simulink model "dtmp_analysis"  (R2025b)
settings: Solver=ode23tb  StartTime=0.0  StopTime=simlength  FixedStep=tc  MaxStep=tc  RelTol=1e-3
values from neighbouring files (symbols this model uses):
  dT_base = 0.4e-3    (= 0.0004)    [init_dtmp_analysis.m]
  N = 40    [init_dtmp_analysis.m]
  tau_dt = Rdt*Cdt    (= 2.706e-06)    [init_dtmp_analysis.m]
  tau_mp = Rmp*Cmp    (= 8.91e-07)    [init_dtmp_analysis.m]
  tc = 1e-7    (= 1e-07)    [init_dtg.m]    (also in init_dtmp_analysis.m)
  Ton_base = 0.333e-6    (= 3.33e-07)    [init_dtmp_analysis.m]
  vin_cmd = 12    [init_dtg.m]    (also in init_dtmp_analysis.m = 15)
libraries: deadtime_with_minimum_pulse_generator x5
settings Model: SimulationMode=accelerator  Creator=dbagn  LastModifiedBy=ltnbda
settings DataIOCC: SaveOutput=off  SignalLogging=off  DSMLogging=off  SaveTime=off  ReturnWorkspaceOutputs=off

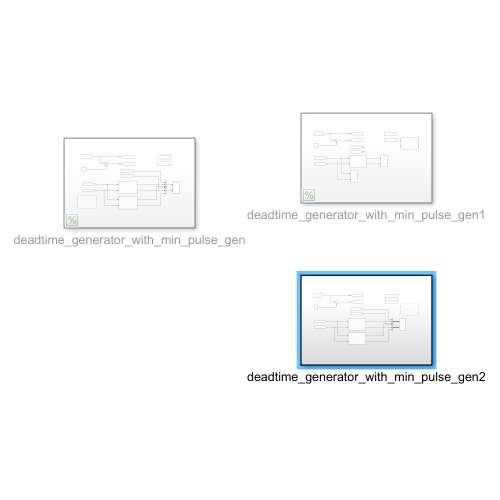
[thumbnail: Simulink's stored preview of the top-level diagram]
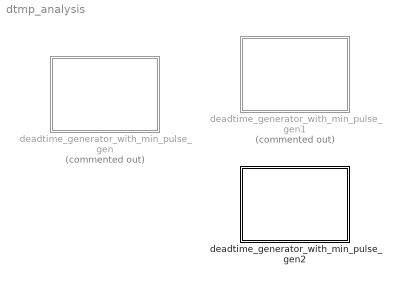
== system dtmp_analysis ==
  deadtime_generator_with_min_pulse_gen : Subsystem  Commented=on
  deadtime_generator_with_min_pulse_gen1 : Subsystem  Commented=on
  deadtime_generator_with_min_pulse_gen2 : Subsystem

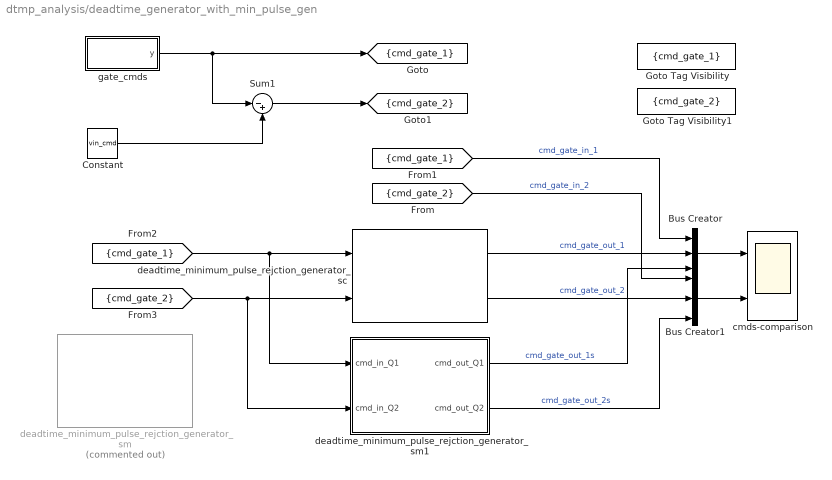
== system dtmp_analysis/deadtime_generator_with_min_pulse_gen ==
  Bus Creator : BusCreator  Inputs=3
  Bus Creator1 : BusCreator  Inputs=3
  Constant : Constant  Value=vin_cmd
  Goto Tag Visibility : GotoTagVisibility  GotoTag=cmd_gate_1
  Goto Tag Visibility1 : GotoTagVisibility  GotoTag=cmd_gate_2
  Sum1 : Sum  Inputs=|-+
  cmds-comparison : Scope  NumInputPorts=2
      settings: SampleTime=tc  ActiveDisplayYMinimum=-1.8749999999999996  ActiveDisplayYMaximum=16.875
  deadtime_minimum_pulse_rejction_generator_sc : deadtime_with_minimum_pulse_generator/deadtime_minimum_pulse_rejction_generator_sc  Vpos_rail_dtg=15  Vneg_rail_dtg=0  Cdt=Cdt  Rdt=Rdt  Cmp=Cmp  Rmp=Rmp
  deadtime_minimum_pulse_rejction_generator_sm : deadtime_with_minimum_pulse_generator/deadtime_minimum_pulse_rejction_generator_sm  Commented=on  Vpos_rail_dtg=12  deadtime=2e-6  minimum_pulse=2e-6
  deadtime_minimum_pulse_rejction_generator_sm1 : Subsystem  mask{Vpos_rail_dtg=15, deadtime=tau_dt, minimum_pulse=tau_mp, tc_m=tc}
      mask prompts: Vpos_rail_dtg "Positive Voltage Rail Supply"; deadtime "DeadTime [s]"; minimum_pulse "Minimum Pulse [s]"; tc_m "tc [s]"
  gate_cmds : Subsystem
  tag scope: cmd_gate_1=scoped, cmd_gate_2=scoped
  wires:
  gate_cmds/1(y) -> [cmd_gate_1], Sum1/1
  [cmd_gate_2] -> Bus Creator1/1  "cmd_gate_in_2"
  [cmd_gate_1] -> Bus Creator/1  "cmd_gate_in_1"
  deadtime_minimum_pulse_rejction_generator_sc/2 -> Bus Creator1/2  "cmd_gate_out_2"
  deadtime_minimum_pulse_rejction_generator_sc/1 -> Bus Creator/2  "cmd_gate_out_1"
  Constant/1 -> Sum1/2
  Sum1/1 -> [cmd_gate_2]
  Bus Creator/1 -> cmds-comparison/1
  Bus Creator1/1 -> cmds-comparison/2
  [cmd_gate_1] -> deadtime_minimum_pulse_rejction_generator_sm1/1(cmd_in_Q1), deadtime_minimum_pulse_rejction_generator_sc/1
  [cmd_gate_2] -> deadtime_minimum_pulse_rejction_generator_sm1/2(cmd_in_Q2), deadtime_minimum_pulse_rejction_generator_sc/2
  deadtime_minimum_pulse_rejction_generator_sm1/1(cmd_out_Q1) -> Bus Creator/3  "cmd_gate_out_1s"
  deadtime_minimum_pulse_rejction_generator_sm1/2(cmd_out_Q2) -> Bus Creator1/3  "cmd_gate_out_2s"

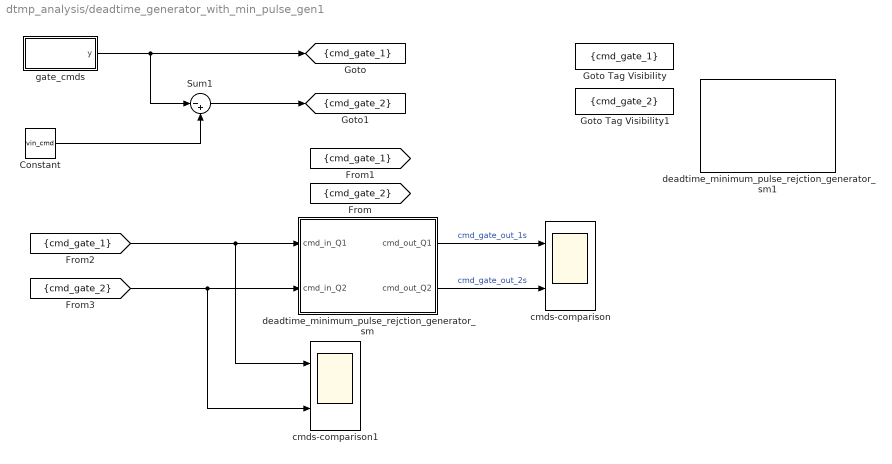
== system dtmp_analysis/deadtime_generator_with_min_pulse_gen1 ==
  Constant : Constant  Value=vin_cmd
  Goto Tag Visibility : GotoTagVisibility  GotoTag=cmd_gate_1
  Goto Tag Visibility1 : GotoTagVisibility  GotoTag=cmd_gate_2
  Sum1 : Sum  Inputs=|-+
  cmds-comparison : Scope  NumInputPorts=2
      settings: SampleTime=tc  ActiveDisplayYMinimum=-1.8749999999999996  ActiveDisplayYMaximum=16.875
  cmds-comparison1 : Scope  NumInputPorts=2
      settings: SampleTime=tc  ActiveDisplayYMinimum=-1.8749999999999996  ActiveDisplayYMaximum=16.875
  deadtime_minimum_pulse_rejction_generator_sm : Subsystem  mask{Vpos_rail_dtg=15, deadtime=tau_dt, minimum_pulse=tau_dt, tc_m=tc}
      mask prompts: Vpos_rail_dtg "Positive Voltage Rail Supply"; deadtime "DeadTime [s]"; minimum_pulse "Minimum Pulse [s]"; tc_m "tc [s]"
  deadtime_minimum_pulse_rejction_generator_sm1 : deadtime_with_minimum_pulse_generator/deadtime_minimum_pulse_rejction_generator_sm  Vpos_rail_dtg=12  deadtime=2e-6  minimum_pulse=2e-6
  gate_cmds : Subsystem
  tag scope: cmd_gate_1=scoped, cmd_gate_2=scoped
  wires:
  [cmd_gate_2] -> deadtime_minimum_pulse_rejction_generator_sm/2(cmd_in_Q2), cmds-comparison1/2
  [cmd_gate_1] -> deadtime_minimum_pulse_rejction_generator_sm/1(cmd_in_Q1), cmds-comparison1/1
  Sum1/1 -> [cmd_gate_2]
  Constant/1 -> Sum1/2
  gate_cmds/1(y) -> Sum1/1, [cmd_gate_1]
  deadtime_minimum_pulse_rejction_generator_sm/1(cmd_out_Q1) -> cmds-comparison/1  "cmd_gate_out_1s"
  deadtime_minimum_pulse_rejction_generator_sm/2(cmd_out_Q2) -> cmds-comparison/2  "cmd_gate_out_2s"

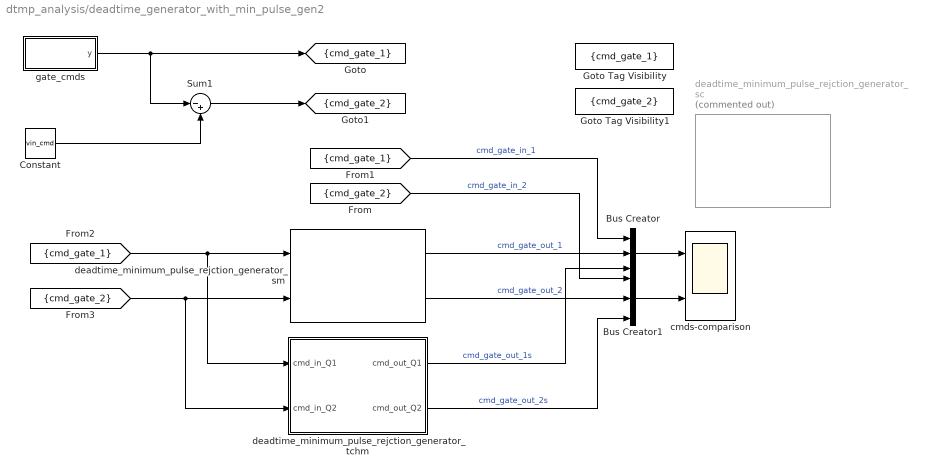
== system dtmp_analysis/deadtime_generator_with_min_pulse_gen2 ==
  Bus Creator : BusCreator  Inputs=3
  Bus Creator1 : BusCreator  Inputs=3
  Constant : Constant  Value=vin_cmd
  Goto Tag Visibility : GotoTagVisibility  GotoTag=cmd_gate_1
  Goto Tag Visibility1 : GotoTagVisibility  GotoTag=cmd_gate_2
  Sum1 : Sum  Inputs=|-+
  cmds-comparison : Scope  NumInputPorts=2
      settings: SampleTime=tc  ActiveDisplayYMinimum=-1.8749999999999996  ActiveDisplayYMaximum=16.875
  deadtime_minimum_pulse_rejction_generator_sc : deadtime_with_minimum_pulse_generator/deadtime_minimum_pulse_rejction_generator_sc  Commented=on  Vpos_rail_dtg=15  Vneg_rail_dtg=0  Cdt=Cdt  Rdt=Rdt  Cmp=Cmp  Rmp=Rmp
  deadtime_minimum_pulse_rejction_generator_sm : deadtime_with_minimum_pulse_generator/deadtime_minimum_pulse_rejction_generator_sm  Vpos_rail_dtg=15  deadtime=tau_dt  minimum_pulse=tau_mp
  deadtime_minimum_pulse_rejction_generator_tchm : Subsystem  mask{Vpos_rail_dtg=15, deadtime=tau_dt, minimum_pulse=tau_mp, tc_m=tc}
      mask prompts: Vpos_rail_dtg "Positive Voltage Rail Supply"; deadtime "DeadTime [s]"; minimum_pulse "Minimum Pulse [s]"; tc_m "tc [s]"
  gate_cmds : Subsystem
  tag scope: cmd_gate_1=scoped, cmd_gate_2=scoped
  wires:
  deadtime_minimum_pulse_rejction_generator_tchm/2(cmd_out_Q2) -> Bus Creator1/3  "cmd_gate_out_2s"
  deadtime_minimum_pulse_rejction_generator_tchm/1(cmd_out_Q1) -> Bus Creator/3  "cmd_gate_out_1s"
  [cmd_gate_2] -> deadtime_minimum_pulse_rejction_generator_sm/2, deadtime_minimum_pulse_rejction_generator_tchm/2(cmd_in_Q2)
  [cmd_gate_1] -> deadtime_minimum_pulse_rejction_generator_sm/1, deadtime_minimum_pulse_rejction_generator_tchm/1(cmd_in_Q1)
  Bus Creator1/1 -> cmds-comparison/2
  Bus Creator/1 -> cmds-comparison/1
  Sum1/1 -> [cmd_gate_2]
  Constant/1 -> Sum1/2
  deadtime_minimum_pulse_rejction_generator_sm/1 -> Bus Creator/2  "cmd_gate_out_1"
  deadtime_minimum_pulse_rejction_generator_sm/2 -> Bus Creator1/2  "cmd_gate_out_2"
  [cmd_gate_1] -> Bus Creator/1  "cmd_gate_in_1"
  [cmd_gate_2] -> Bus Creator1/1  "cmd_gate_in_2"
  gate_cmds/1(y) -> Sum1/1, [cmd_gate_1]

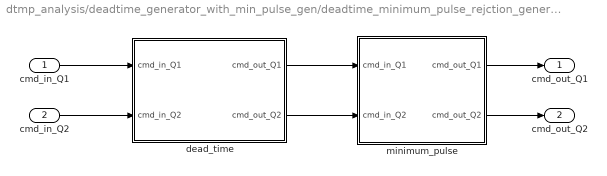
== system dtmp_analysis/deadtime_generator_with_min_pulse_gen/deadtime_minimum_pulse_rejction_generator_sm1 ==
  cmd_in_Q1 : Inport
  cmd_in_Q2 : Inport  Port=2
  dead_time : Subsystem
  minimum_pulse : Subsystem
  cmd_out_Q1 : Outport
  cmd_out_Q2 : Outport  Port=2
  wires:
  cmd_in_Q1/1 -> dead_time/1(cmd_in_Q1)
  cmd_in_Q2/1 -> dead_time/2(cmd_in_Q2)
  dead_time/1(cmd_out_Q1) -> minimum_pulse/1(cmd_in_Q1)
  dead_time/2(cmd_out_Q2) -> minimum_pulse/2(cmd_in_Q2)
  minimum_pulse/1(cmd_out_Q1) -> cmd_out_Q1/1
  minimum_pulse/2(cmd_out_Q2) -> cmd_out_Q2/1

== system dtmp_analysis/deadtime_generator_with_min_pulse_gen/gate_cmds ==
  Clock : Clock
  MATLAB Function : MATLAB Function  TreatAsAtomicUnit=on
  y : Outport
  wires:
  MATLAB Function/1(y) -> y/1
  Clock/1 -> MATLAB Function/1(time)

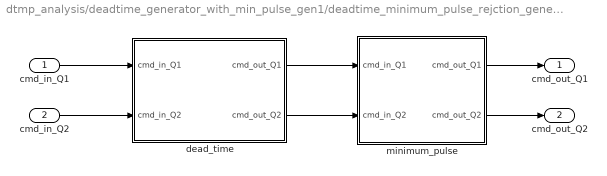
== system dtmp_analysis/deadtime_generator_with_min_pulse_gen1/deadtime_minimum_pulse_rejction_generator_sm ==
  cmd_in_Q1 : Inport
  cmd_in_Q2 : Inport  Port=2
  dead_time : Subsystem
  minimum_pulse : Subsystem
  cmd_out_Q1 : Outport
  cmd_out_Q2 : Outport  Port=2
  wires:
  cmd_in_Q1/1 -> dead_time/1(cmd_in_Q1)
  cmd_in_Q2/1 -> dead_time/2(cmd_in_Q2)
  dead_time/1(cmd_out_Q1) -> minimum_pulse/1(cmd_in_Q1)
  dead_time/2(cmd_out_Q2) -> minimum_pulse/2(cmd_in_Q2)
  minimum_pulse/1(cmd_out_Q1) -> cmd_out_Q1/1
  minimum_pulse/2(cmd_out_Q2) -> cmd_out_Q2/1

== system dtmp_analysis/deadtime_generator_with_min_pulse_gen1/gate_cmds ==
  Clock : Clock
  MATLAB Function : MATLAB Function  TreatAsAtomicUnit=on  SystemSampleTime=tc
  y : Outport
  wires:
  Clock/1 -> MATLAB Function/1(time)
  MATLAB Function/1(y) -> y/1

== system dtmp_analysis/deadtime_generator_with_min_pulse_gen2/deadtime_minimum_pulse_rejction_generator_tchm ==
  cmd_in_Q1 : Inport
  cmd_in_Q2 : Inport  Port=2
  dead_time : Subsystem
  minimum_pulse : Subsystem
  cmd_out_Q1 : Outport
  cmd_out_Q2 : Outport  Port=2
  wires:
  minimum_pulse/2(cmd_out_Q2) -> cmd_out_Q2/1
  minimum_pulse/1(cmd_out_Q1) -> cmd_out_Q1/1
  dead_time/2(cmd_out_Q2) -> minimum_pulse/2(cmd_in_Q2)
  dead_time/1(cmd_out_Q1) -> minimum_pulse/1(cmd_in_Q1)
  cmd_in_Q2/1 -> dead_time/2(cmd_in_Q2)
  cmd_in_Q1/1 -> dead_time/1(cmd_in_Q1)

== system dtmp_analysis/deadtime_generator_with_min_pulse_gen2/gate_cmds ==
  Clock : Clock
  MATLAB Function : MATLAB Function  TreatAsAtomicUnit=on
  y : Outport
  wires:
  Clock/1 -> MATLAB Function/1(time)
  MATLAB Function/1(y) -> y/1

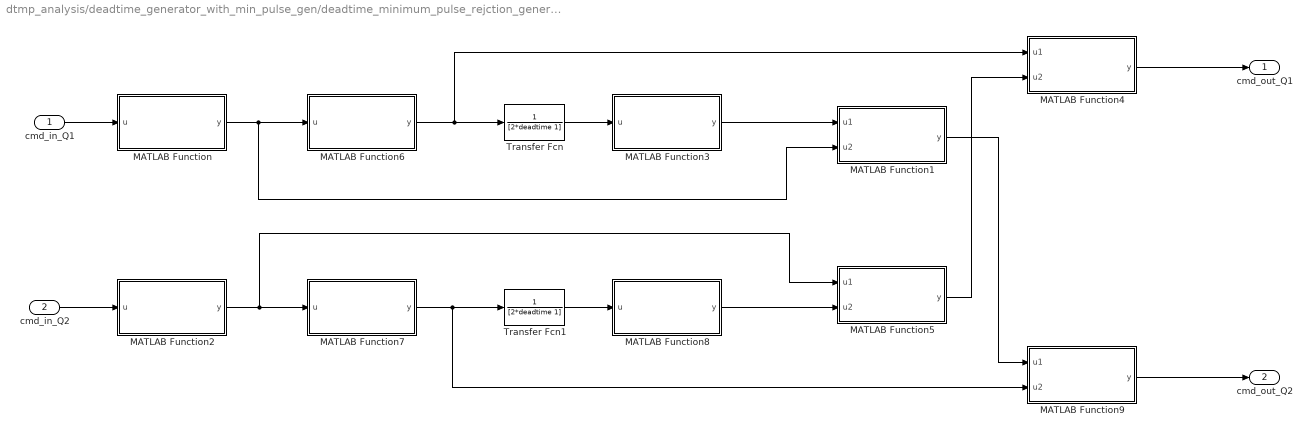
== system dtmp_analysis/deadtime_generator_with_min_pulse_gen/deadtime_minimum_pulse_rejction_generator_sm1/dead_time ==
  cmd_in_Q1 : Inport
  cmd_in_Q2 : Inport  Port=2
  MATLAB Function : MATLAB Function  TreatAsAtomicUnit=on  SystemSampleTime=tc_m
  MATLAB Function1 : MATLAB Function  TreatAsAtomicUnit=on  SystemSampleTime=tc_m
  MATLAB Function2 : MATLAB Function  TreatAsAtomicUnit=on  SystemSampleTime=tc_m
  MATLAB Function3 : MATLAB Function  TreatAsAtomicUnit=on  SystemSampleTime=tc_m
  MATLAB Function4 : MATLAB Function  TreatAsAtomicUnit=on  SystemSampleTime=tc_m
  MATLAB Function5 : MATLAB Function  TreatAsAtomicUnit=on  SystemSampleTime=tc_m
  MATLAB Function6 : MATLAB Function  TreatAsAtomicUnit=on  SystemSampleTime=tc_m
  MATLAB Function7 : MATLAB Function  TreatAsAtomicUnit=on  SystemSampleTime=tc_m
  MATLAB Function8 : MATLAB Function  TreatAsAtomicUnit=on  SystemSampleTime=tc_m
  MATLAB Function9 : MATLAB Function  TreatAsAtomicUnit=on  SystemSampleTime=tc_m
  Transfer Fcn : TransferFcn  Denominator=[2*deadtime 1]
  Transfer Fcn1 : TransferFcn  Denominator=[2*deadtime 1]
  cmd_out_Q1 : Outport
  cmd_out_Q2 : Outport  Port=2
  wires:
  MATLAB Function8/1(y) -> MATLAB Function5/2(u2)
  MATLAB Function3/1(y) -> MATLAB Function1/1(u1)
  MATLAB Function6/1(y) -> MATLAB Function4/1(u1), Transfer Fcn/1
  MATLAB Function7/1(y) -> MATLAB Function9/2(u2), Transfer Fcn1/1
  MATLAB Function2/1(y) -> MATLAB Function7/1(u), MATLAB Function5/1(u1)
  cmd_in_Q2/1 -> MATLAB Function2/1(u)
  MATLAB Function1/1(y) -> MATLAB Function9/1(u1)
  Transfer Fcn1/1 -> MATLAB Function8/1(u)
  cmd_in_Q1/1 -> MATLAB Function/1(u)
  Transfer Fcn/1 -> MATLAB Function3/1(u)
  MATLAB Function5/1(y) -> MATLAB Function4/2(u2)
  MATLAB Function4/1(y) -> cmd_out_Q1/1
  MATLAB Function9/1(y) -> cmd_out_Q2/1
  MATLAB Function/1(y) -> MATLAB Function6/1(u), MATLAB Function1/2(u2)

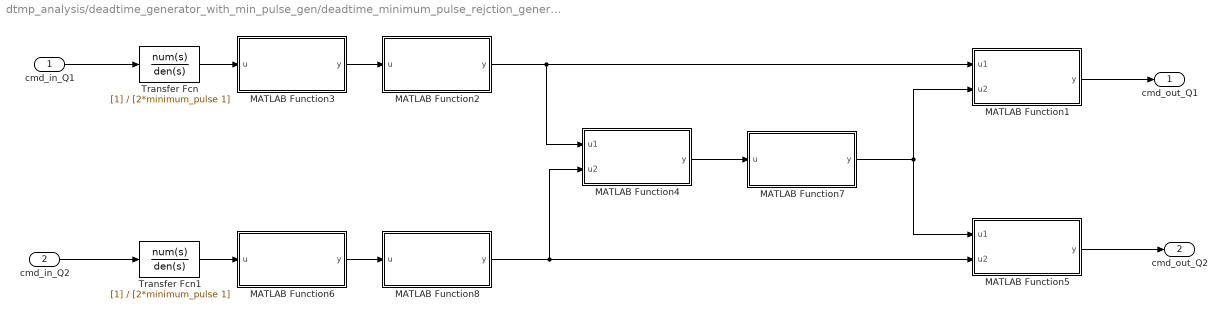
== system dtmp_analysis/deadtime_generator_with_min_pulse_gen/deadtime_minimum_pulse_rejction_generator_sm1/minimum_pulse ==
  cmd_in_Q1 : Inport
  cmd_in_Q2 : Inport  Port=2
  MATLAB Function1 : MATLAB Function  TreatAsAtomicUnit=on  SystemSampleTime=tc_m
  MATLAB Function2 : MATLAB Function  TreatAsAtomicUnit=on  SystemSampleTime=tc_m
  MATLAB Function3 : MATLAB Function  TreatAsAtomicUnit=on  SystemSampleTime=tc_m
  MATLAB Function4 : MATLAB Function  TreatAsAtomicUnit=on  SystemSampleTime=tc_m
  MATLAB Function5 : MATLAB Function  TreatAsAtomicUnit=on  SystemSampleTime=tc_m
  MATLAB Function6 : MATLAB Function  TreatAsAtomicUnit=on  SystemSampleTime=tc_m
  MATLAB Function7 : MATLAB Function  TreatAsAtomicUnit=on  SystemSampleTime=tc_m
  MATLAB Function8 : MATLAB Function  TreatAsAtomicUnit=on  SystemSampleTime=tc_m
  Transfer Fcn : TransferFcn  Denominator=[2*minimum_pulse 1]
  Transfer Fcn1 : TransferFcn  Denominator=[2*minimum_pulse 1]
  cmd_out_Q1 : Outport
  cmd_out_Q2 : Outport  Port=2
  wires:
  MATLAB Function4/1(y) -> MATLAB Function7/1(u)
  Transfer Fcn1/1 -> MATLAB Function6/1(u)
  MATLAB Function3/1(y) -> MATLAB Function2/1(u)
  cmd_in_Q2/1 -> Transfer Fcn1/1
  cmd_in_Q1/1 -> Transfer Fcn/1
  Transfer Fcn/1 -> MATLAB Function3/1(u)
  MATLAB Function1/1(y) -> cmd_out_Q1/1
  MATLAB Function5/1(y) -> cmd_out_Q2/1
  MATLAB Function2/1(y) -> MATLAB Function1/1(u1), MATLAB Function4/1(u1)
  MATLAB Function6/1(y) -> MATLAB Function8/1(u)
  MATLAB Function8/1(y) -> MATLAB Function5/2(u2), MATLAB Function4/2(u2)
  MATLAB Function7/1(y) -> MATLAB Function1/2(u2), MATLAB Function5/1(u1)

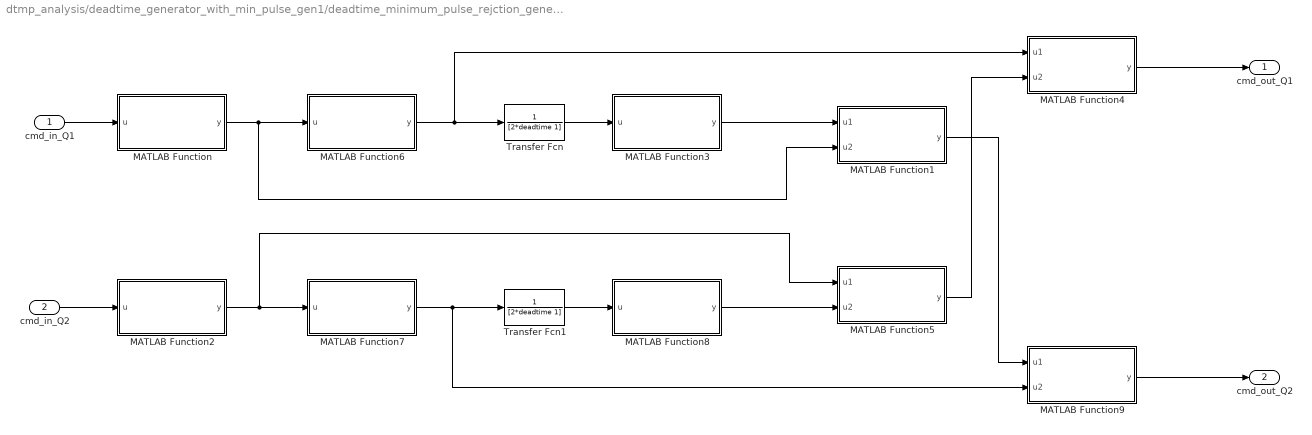
== system dtmp_analysis/deadtime_generator_with_min_pulse_gen1/deadtime_minimum_pulse_rejction_generator_sm/dead_time ==
  cmd_in_Q1 : Inport
  cmd_in_Q2 : Inport  Port=2
  MATLAB Function : MATLAB Function  TreatAsAtomicUnit=on  SystemSampleTime=tc_m
  MATLAB Function1 : MATLAB Function  TreatAsAtomicUnit=on  SystemSampleTime=tc_m
  MATLAB Function2 : MATLAB Function  TreatAsAtomicUnit=on  SystemSampleTime=tc_m
  MATLAB Function3 : MATLAB Function  TreatAsAtomicUnit=on  SystemSampleTime=tc_m
  MATLAB Function4 : MATLAB Function  TreatAsAtomicUnit=on  SystemSampleTime=tc_m
  MATLAB Function5 : MATLAB Function  TreatAsAtomicUnit=on  SystemSampleTime=tc_m
  MATLAB Function6 : MATLAB Function  TreatAsAtomicUnit=on  SystemSampleTime=tc_m
  MATLAB Function7 : MATLAB Function  TreatAsAtomicUnit=on  SystemSampleTime=tc_m
  MATLAB Function8 : MATLAB Function  TreatAsAtomicUnit=on  SystemSampleTime=tc_m
  MATLAB Function9 : MATLAB Function  TreatAsAtomicUnit=on  SystemSampleTime=tc_m
  Transfer Fcn : TransferFcn  Denominator=[2*deadtime 1]
  Transfer Fcn1 : TransferFcn  Denominator=[2*deadtime 1]
  cmd_out_Q1 : Outport
  cmd_out_Q2 : Outport  Port=2
  wires:
  MATLAB Function8/1(y) -> MATLAB Function5/2(u2)
  MATLAB Function3/1(y) -> MATLAB Function1/1(u1)
  MATLAB Function6/1(y) -> MATLAB Function4/1(u1), Transfer Fcn/1
  MATLAB Function7/1(y) -> MATLAB Function9/2(u2), Transfer Fcn1/1
  MATLAB Function2/1(y) -> MATLAB Function7/1(u), MATLAB Function5/1(u1)
  cmd_in_Q2/1 -> MATLAB Function2/1(u)
  MATLAB Function1/1(y) -> MATLAB Function9/1(u1)
  Transfer Fcn1/1 -> MATLAB Function8/1(u)
  cmd_in_Q1/1 -> MATLAB Function/1(u)
  Transfer Fcn/1 -> MATLAB Function3/1(u)
  MATLAB Function5/1(y) -> MATLAB Function4/2(u2)
  MATLAB Function4/1(y) -> cmd_out_Q1/1
  MATLAB Function9/1(y) -> cmd_out_Q2/1
  MATLAB Function/1(y) -> MATLAB Function6/1(u), MATLAB Function1/2(u2)

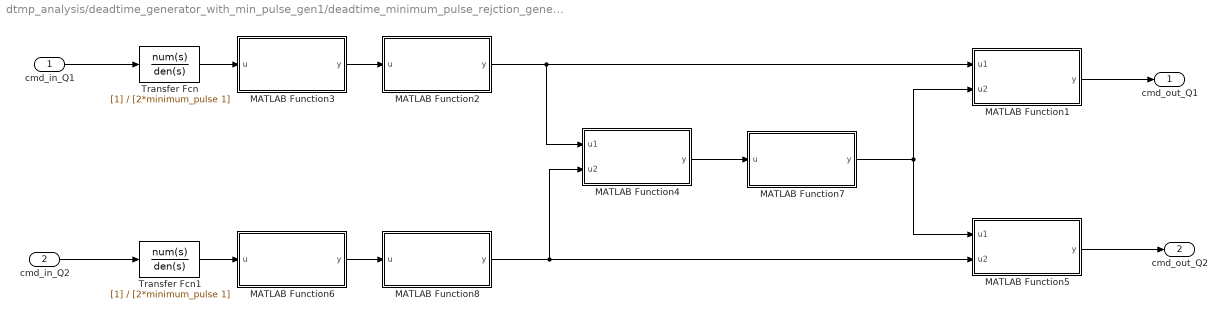
== system dtmp_analysis/deadtime_generator_with_min_pulse_gen1/deadtime_minimum_pulse_rejction_generator_sm/minimum_pulse ==
  cmd_in_Q1 : Inport
  cmd_in_Q2 : Inport  Port=2
  MATLAB Function1 : MATLAB Function  TreatAsAtomicUnit=on  SystemSampleTime=tc_m
  MATLAB Function2 : MATLAB Function  TreatAsAtomicUnit=on  SystemSampleTime=tc_m
  MATLAB Function3 : MATLAB Function  TreatAsAtomicUnit=on  SystemSampleTime=tc_m
  MATLAB Function4 : MATLAB Function  TreatAsAtomicUnit=on  SystemSampleTime=tc_m
  MATLAB Function5 : MATLAB Function  TreatAsAtomicUnit=on  SystemSampleTime=tc_m
  MATLAB Function6 : MATLAB Function  TreatAsAtomicUnit=on  SystemSampleTime=tc_m
  MATLAB Function7 : MATLAB Function  TreatAsAtomicUnit=on  SystemSampleTime=tc_m
  MATLAB Function8 : MATLAB Function  TreatAsAtomicUnit=on  SystemSampleTime=tc_m
  Transfer Fcn : TransferFcn  Denominator=[2*minimum_pulse 1]
  Transfer Fcn1 : TransferFcn  Denominator=[2*minimum_pulse 1]
  cmd_out_Q1 : Outport
  cmd_out_Q2 : Outport  Port=2
  wires:
  MATLAB Function4/1(y) -> MATLAB Function7/1(u)
  Transfer Fcn1/1 -> MATLAB Function6/1(u)
  MATLAB Function3/1(y) -> MATLAB Function2/1(u)
  cmd_in_Q2/1 -> Transfer Fcn1/1
  cmd_in_Q1/1 -> Transfer Fcn/1
  Transfer Fcn/1 -> MATLAB Function3/1(u)
  MATLAB Function1/1(y) -> cmd_out_Q1/1
  MATLAB Function5/1(y) -> cmd_out_Q2/1
  MATLAB Function2/1(y) -> MATLAB Function1/1(u1), MATLAB Function4/1(u1)
  MATLAB Function6/1(y) -> MATLAB Function8/1(u)
  MATLAB Function8/1(y) -> MATLAB Function5/2(u2), MATLAB Function4/2(u2)
  MATLAB Function7/1(y) -> MATLAB Function1/2(u2), MATLAB Function5/1(u1)

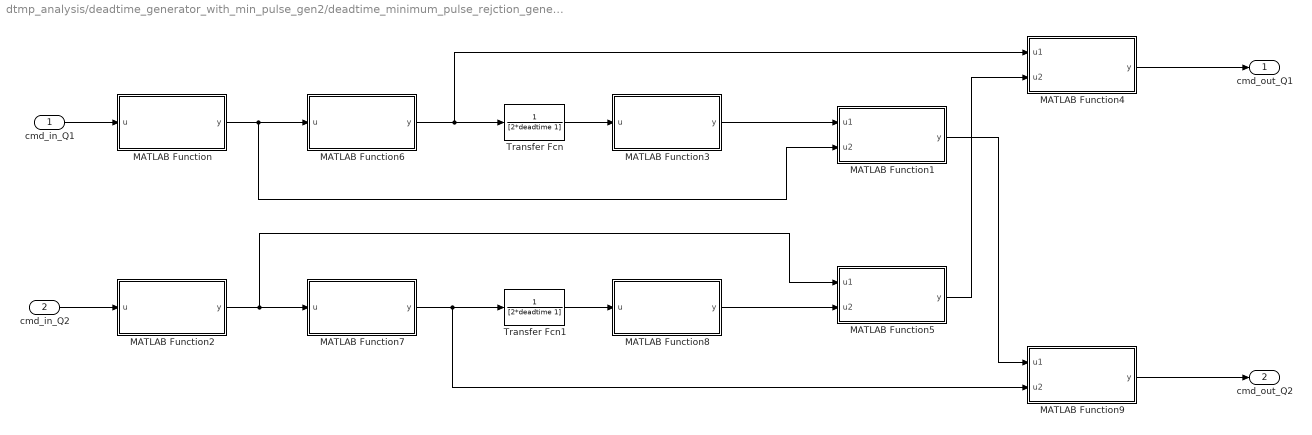
== system dtmp_analysis/deadtime_generator_with_min_pulse_gen2/deadtime_minimum_pulse_rejction_generator_tchm/dead_time ==
  cmd_in_Q1 : Inport
  cmd_in_Q2 : Inport  Port=2
  MATLAB Function : MATLAB Function  TreatAsAtomicUnit=on  SystemSampleTime=tc_m
  MATLAB Function1 : MATLAB Function  TreatAsAtomicUnit=on  SystemSampleTime=tc_m
  MATLAB Function2 : MATLAB Function  TreatAsAtomicUnit=on  SystemSampleTime=tc_m
  MATLAB Function3 : MATLAB Function  TreatAsAtomicUnit=on  SystemSampleTime=tc_m
  MATLAB Function4 : MATLAB Function  TreatAsAtomicUnit=on  SystemSampleTime=tc_m
  MATLAB Function5 : MATLAB Function  TreatAsAtomicUnit=on  SystemSampleTime=tc_m
  MATLAB Function6 : MATLAB Function  TreatAsAtomicUnit=on  SystemSampleTime=tc_m
  MATLAB Function7 : MATLAB Function  TreatAsAtomicUnit=on  SystemSampleTime=tc_m
  MATLAB Function8 : MATLAB Function  TreatAsAtomicUnit=on  SystemSampleTime=tc_m
  MATLAB Function9 : MATLAB Function  TreatAsAtomicUnit=on  SystemSampleTime=tc_m
  Transfer Fcn : TransferFcn  Denominator=[2*deadtime 1]
  Transfer Fcn1 : TransferFcn  Denominator=[2*deadtime 1]
  cmd_out_Q1 : Outport
  cmd_out_Q2 : Outport  Port=2
  wires:
  MATLAB Function/1(y) -> MATLAB Function1/2(u2), MATLAB Function6/1(u)
  MATLAB Function9/1(y) -> cmd_out_Q2/1
  MATLAB Function4/1(y) -> cmd_out_Q1/1
  MATLAB Function5/1(y) -> MATLAB Function4/2(u2)
  Transfer Fcn/1 -> MATLAB Function3/1(u)
  cmd_in_Q1/1 -> MATLAB Function/1(u)
  Transfer Fcn1/1 -> MATLAB Function8/1(u)
  MATLAB Function1/1(y) -> MATLAB Function9/1(u1)
  cmd_in_Q2/1 -> MATLAB Function2/1(u)
  MATLAB Function2/1(y) -> MATLAB Function5/1(u1), MATLAB Function7/1(u)
  MATLAB Function7/1(y) -> Transfer Fcn1/1, MATLAB Function9/2(u2)
  MATLAB Function6/1(y) -> Transfer Fcn/1, MATLAB Function4/1(u1)
  MATLAB Function3/1(y) -> MATLAB Function1/1(u1)
  MATLAB Function8/1(y) -> MATLAB Function5/2(u2)

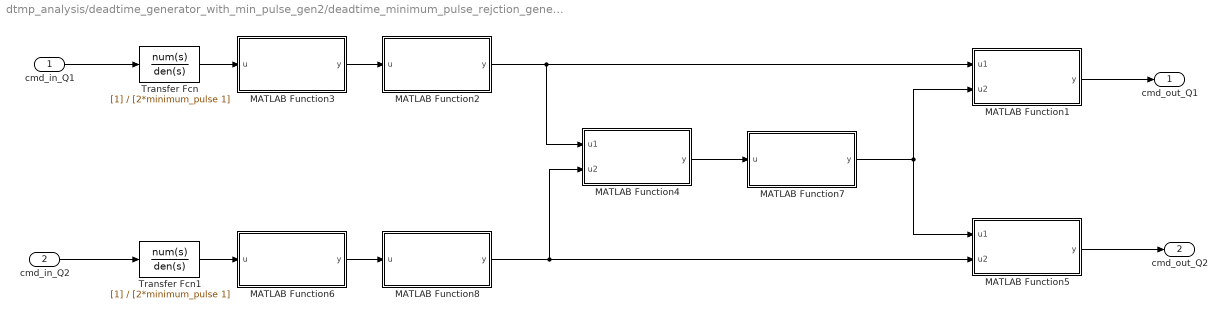
== system dtmp_analysis/deadtime_generator_with_min_pulse_gen2/deadtime_minimum_pulse_rejction_generator_tchm/minimum_pulse ==
  cmd_in_Q1 : Inport
  cmd_in_Q2 : Inport  Port=2
  MATLAB Function1 : MATLAB Function  TreatAsAtomicUnit=on  SystemSampleTime=tc_m
  MATLAB Function2 : MATLAB Function  TreatAsAtomicUnit=on  SystemSampleTime=tc_m
  MATLAB Function3 : MATLAB Function  TreatAsAtomicUnit=on  SystemSampleTime=tc_m
  MATLAB Function4 : MATLAB Function  TreatAsAtomicUnit=on  SystemSampleTime=tc_m
  MATLAB Function5 : MATLAB Function  TreatAsAtomicUnit=on  SystemSampleTime=tc_m
  MATLAB Function6 : MATLAB Function  TreatAsAtomicUnit=on  SystemSampleTime=tc_m
  MATLAB Function7 : MATLAB Function  TreatAsAtomicUnit=on  SystemSampleTime=tc_m
  MATLAB Function8 : MATLAB Function  TreatAsAtomicUnit=on  SystemSampleTime=tc_m
  Transfer Fcn : TransferFcn  Denominator=[2*minimum_pulse 1]
  Transfer Fcn1 : TransferFcn  Denominator=[2*minimum_pulse 1]
  cmd_out_Q1 : Outport
  cmd_out_Q2 : Outport  Port=2
  wires:
  MATLAB Function7/1(y) -> MATLAB Function5/1(u1), MATLAB Function1/2(u2)
  MATLAB Function8/1(y) -> MATLAB Function4/2(u2), MATLAB Function5/2(u2)
  MATLAB Function6/1(y) -> MATLAB Function8/1(u)
  MATLAB Function2/1(y) -> MATLAB Function4/1(u1), MATLAB Function1/1(u1)
  MATLAB Function5/1(y) -> cmd_out_Q2/1
  MATLAB Function1/1(y) -> cmd_out_Q1/1
  Transfer Fcn/1 -> MATLAB Function3/1(u)
  cmd_in_Q1/1 -> Transfer Fcn/1
  cmd_in_Q2/1 -> Transfer Fcn1/1
  MATLAB Function3/1(y) -> MATLAB Function2/1(u)
  Transfer Fcn1/1 -> MATLAB Function6/1(u)
  MATLAB Function4/1(y) -> MATLAB Function7/1(u)

== matlab function dtmp_analysis/deadtime_generator_with_min_pulse_gen/deadtime_minimum_pulse_rejction_generator_sm1/dead_time/MATLAB Function ==
  data: u input; y output; Vpos_rail_dtg parameter
function y = tschimitt_not_cmos(u, Vpos_rail_dtg)

persistent y_old

if isempty(y_old)
    y_old = 0;
end

vth1 = Vpos_rail_dtg*0.75;
vth2 = Vpos_rail_dtg*0.25;

if u > vth1
    y = 0;
    y_old = y;
elseif u < vth2
    y = Vpos_rail_dtg;
    y_old = y;
else
    y = y_old;
end

== matlab function dtmp_analysis/deadtime_generator_with_min_pulse_gen/deadtime_minimum_pulse_rejction_generator_sm1/dead_time/MATLAB Function1 ==
  data: u1 input; u2 input; y output; Vpos_rail_dtg parameter
function y = and_cmos(u1, u2, Vpos_rail_dtg)

vth = Vpos_rail_dtg/2;

if (u1 > vth && u2 > vth)
    y = Vpos_rail_dtg;
else
    y = 0;
end

== matlab function dtmp_analysis/deadtime_generator_with_min_pulse_gen/deadtime_minimum_pulse_rejction_generator_sm1/dead_time/MATLAB Function2 ==
  data: u input; y output; Vpos_rail_dtg parameter
function y = tschimitt_not_cmos(u, Vpos_rail_dtg)

persistent y_old

if isempty(y_old)
    y_old = 0;
end

vth1 = Vpos_rail_dtg*0.75;
vth2 = Vpos_rail_dtg*0.25;

if u > vth1
    y = 0;
    y_old = y;
elseif u < vth2
    y = Vpos_rail_dtg;
    y_old = y;
else
    y = y_old;
end

== matlab function dtmp_analysis/deadtime_generator_with_min_pulse_gen/deadtime_minimum_pulse_rejction_generator_sm1/dead_time/MATLAB Function3 ==
  data: u input; y output; Vpos_rail_dtg parameter
function y = tschimitt_not_cmos(u, Vpos_rail_dtg)

persistent y_old

if isempty(y_old)
    y_old = 0;
end

vth1 = Vpos_rail_dtg*0.75;
vth2 = Vpos_rail_dtg*0.25;

if u > vth1
    y = 0;
    y_old = y;
elseif u < vth2
    y = Vpos_rail_dtg;
    y_old = y;
else
    y = y_old;
end

== matlab function dtmp_analysis/deadtime_generator_with_min_pulse_gen/deadtime_minimum_pulse_rejction_generator_sm1/dead_time/MATLAB Function4 ==
  data: u1 input; u2 input; y output; Vpos_rail_dtg parameter
function y = and_cmos(u1, u2, Vpos_rail_dtg)

vth = Vpos_rail_dtg/2;

if (u1 > vth && u2 > vth)
    y = Vpos_rail_dtg;
else
    y = 0;
end

== matlab function dtmp_analysis/deadtime_generator_with_min_pulse_gen/deadtime_minimum_pulse_rejction_generator_sm1/dead_time/MATLAB Function5 ==
  data: u1 input; u2 input; y output; Vpos_rail_dtg parameter
function y = and_cmos(u1, u2, Vpos_rail_dtg)

vth = Vpos_rail_dtg/2;

if (u1 > vth && u2 > vth)
    y = Vpos_rail_dtg;
else
    y = 0;
end

== matlab function dtmp_analysis/deadtime_generator_with_min_pulse_gen/deadtime_minimum_pulse_rejction_generator_sm1/dead_time/MATLAB Function6 ==
  data: u input; y output; Vpos_rail_dtg parameter
function y = tschimitt_not_cmos(u, Vpos_rail_dtg)

persistent y_old

if isempty(y_old)
    y_old = 0;
end

vth1 = Vpos_rail_dtg*0.75;
vth2 = Vpos_rail_dtg*0.25;

if u > vth1
    y = 0;
    y_old = y;
elseif u < vth2
    y = Vpos_rail_dtg;
    y_old = y;
else
    y = y_old;
end

== matlab function dtmp_analysis/deadtime_generator_with_min_pulse_gen/deadtime_minimum_pulse_rejction_generator_sm1/dead_time/MATLAB Function7 ==
  data: u input; y output; Vpos_rail_dtg parameter
function y = tschimitt_not_cmos(u, Vpos_rail_dtg)

persistent y_old

if isempty(y_old)
    y_old = 0;
end

vth1 = Vpos_rail_dtg*0.75;
vth2 = Vpos_rail_dtg*0.25;

if u > vth1
    y = 0;
    y_old = y;
elseif u < vth2
    y = Vpos_rail_dtg;
    y_old = y;
else
    y = y_old;
end

== matlab function dtmp_analysis/deadtime_generator_with_min_pulse_gen1/deadtime_minimum_pulse_rejction_generator_sm/dead_time/MATLAB Function ==
  data: u input; y output; Vpos_rail_dtg parameter
function y = tschimitt_not_cmos(u, Vpos_rail_dtg)

persistent y_old

if isempty(y_old)
    y_old = 0;
end

vth1 = Vpos_rail_dtg*0.75;
vth2 = Vpos_rail_dtg*0.25;

if u > vth1
    y = 0;
    y_old = y;
elseif u < vth2
    y = Vpos_rail_dtg;
    y_old = y;
else
    y = y_old;
end

== matlab function dtmp_analysis/deadtime_generator_with_min_pulse_gen1/deadtime_minimum_pulse_rejction_generator_sm/dead_time/MATLAB Function1 ==
  data: u1 input; u2 input; y output; Vpos_rail_dtg parameter
function y = and_cmos(u1, u2, Vpos_rail_dtg)

vth = Vpos_rail_dtg/2;

if (u1 > vth && u2 > vth)
    y = Vpos_rail_dtg;
else
    y = 0;
end

== matlab function dtmp_analysis/deadtime_generator_with_min_pulse_gen1/deadtime_minimum_pulse_rejction_generator_sm/dead_time/MATLAB Function2 ==
  data: u input; y output; Vpos_rail_dtg parameter
function y = tschimitt_not_cmos(u, Vpos_rail_dtg)

persistent y_old

if isempty(y_old)
    y_old = 0;
end

vth1 = Vpos_rail_dtg*0.75;
vth2 = Vpos_rail_dtg*0.25;

if u > vth1
    y = 0;
    y_old = y;
elseif u < vth2
    y = Vpos_rail_dtg;
    y_old = y;
else
    y = y_old;
end

== matlab function dtmp_analysis/deadtime_generator_with_min_pulse_gen/deadtime_minimum_pulse_rejction_generator_sm1/dead_time/MATLAB Function8 ==
  data: u input; y output; Vpos_rail_dtg parameter
function y = tschimitt_not_cmos(u, Vpos_rail_dtg)

persistent y_old

if isempty(y_old)
    y_old = 0;
end

vth1 = Vpos_rail_dtg*0.75;
vth2 = Vpos_rail_dtg*0.25;

if u > vth1
    y = 0;
    y_old = y;
elseif u < vth2
    y = Vpos_rail_dtg;
    y_old = y;
else
    y = y_old;
end

== matlab function dtmp_analysis/deadtime_generator_with_min_pulse_gen/deadtime_minimum_pulse_rejction_generator_sm1/dead_time/MATLAB Function9 ==
  data: u1 input; u2 input; y output; Vpos_rail_dtg parameter
function y = and_cmos(u1, u2, Vpos_rail_dtg)

vth = Vpos_rail_dtg/2;

if (u1 > vth && u2 > vth)
    y = Vpos_rail_dtg;
else
    y = 0;
end

== matlab function dtmp_analysis/deadtime_generator_with_min_pulse_gen1/deadtime_minimum_pulse_rejction_generator_sm/dead_time/MATLAB Function4 ==
  data: u1 input; u2 input; y output; Vpos_rail_dtg parameter
function y = and_cmos(u1, u2, Vpos_rail_dtg)

vth = Vpos_rail_dtg/2;

if (u1 > vth && u2 > vth)
    y = Vpos_rail_dtg;
else
    y = 0;
end

== matlab function dtmp_analysis/deadtime_generator_with_min_pulse_gen1/deadtime_minimum_pulse_rejction_generator_sm/dead_time/MATLAB Function5 ==
  data: u1 input; u2 input; y output; Vpos_rail_dtg parameter
function y = and_cmos(u1, u2, Vpos_rail_dtg)

vth = Vpos_rail_dtg/2;

if (u1 > vth && u2 > vth)
    y = Vpos_rail_dtg;
else
    y = 0;
end

== matlab function dtmp_analysis/deadtime_generator_with_min_pulse_gen/deadtime_minimum_pulse_rejction_generator_sm1/minimum_pulse/MATLAB Function1 ==
  data: u1 input; u2 input; y output; Vpos_rail_dtg parameter
function y = and_cmos(u1, u2, Vpos_rail_dtg)

vth = Vpos_rail_dtg/2;

if (u1 > vth && u2 > vth)
    y = Vpos_rail_dtg;
else
    y = 0;
end

== matlab function dtmp_analysis/deadtime_generator_with_min_pulse_gen/deadtime_minimum_pulse_rejction_generator_sm1/minimum_pulse/MATLAB Function2 ==
  data: u input; y output; Vpos_rail_dtg parameter
function y = tschimitt_not_cmos(u, Vpos_rail_dtg)

persistent y_old

if isempty(y_old)
    y_old = 0;
end

vth1 = Vpos_rail_dtg*0.75;
vth2 = Vpos_rail_dtg*0.25;

if u > vth1
    y = 0;
    y_old = y;
elseif u < vth2
    y = Vpos_rail_dtg;
    y_old = y;
else
    y = y_old;
end

== matlab function dtmp_analysis/deadtime_generator_with_min_pulse_gen/deadtime_minimum_pulse_rejction_generator_sm1/minimum_pulse/MATLAB Function3 ==
  data: u input; y output; Vpos_rail_dtg parameter
function y = tschimitt_not_cmos(u, Vpos_rail_dtg)

persistent y_old

if isempty(y_old)
    y_old = 0;
end

vth1 = Vpos_rail_dtg*0.75;
vth2 = Vpos_rail_dtg*0.25;

if u > vth1
    y = 0;
    y_old = y;
elseif u < vth2
    y = Vpos_rail_dtg;
    y_old = y;
else
    y = y_old;
end

== matlab function dtmp_analysis/deadtime_generator_with_min_pulse_gen1/deadtime_minimum_pulse_rejction_generator_sm/dead_time/MATLAB Function9 ==
  data: u1 input; u2 input; y output; Vpos_rail_dtg parameter
function y = and_cmos(u1, u2, Vpos_rail_dtg)

vth = Vpos_rail_dtg/2;

if (u1 > vth && u2 > vth)
    y = Vpos_rail_dtg;
else
    y = 0;
end

== matlab function dtmp_analysis/deadtime_generator_with_min_pulse_gen1/deadtime_minimum_pulse_rejction_generator_sm/minimum_pulse/MATLAB Function1 ==
  data: u1 input; u2 input; y output; Vpos_rail_dtg parameter
function y = and_cmos(u1, u2, Vpos_rail_dtg)

vth = Vpos_rail_dtg/2;

if (u1 > vth && u2 > vth)
    y = Vpos_rail_dtg;
else
    y = 0;
end

== matlab function dtmp_analysis/deadtime_generator_with_min_pulse_gen1/deadtime_minimum_pulse_rejction_generator_sm/dead_time/MATLAB Function6 ==
  data: u input; y output; Vpos_rail_dtg parameter
function y = tschimitt_not_cmos(u, Vpos_rail_dtg)

persistent y_old

if isempty(y_old)
    y_old = 0;
end

vth1 = Vpos_rail_dtg*0.75;
vth2 = Vpos_rail_dtg*0.25;

if u > vth1
    y = 0;
    y_old = y;
elseif u < vth2
    y = Vpos_rail_dtg;
    y_old = y;
else
    y = y_old;
end

== matlab function dtmp_analysis/deadtime_generator_with_min_pulse_gen/deadtime_minimum_pulse_rejction_generator_sm1/minimum_pulse/MATLAB Function4 ==
  data: u1 input; u2 input; y output; Vpos_rail_dtg parameter
function y = and_cmos(u1, u2, Vpos_rail_dtg)

vth = Vpos_rail_dtg/2;

if (u1 > vth && u2 > vth)
    y = Vpos_rail_dtg;
else
    y = 0;
end

== matlab function dtmp_analysis/deadtime_generator_with_min_pulse_gen/deadtime_minimum_pulse_rejction_generator_sm1/minimum_pulse/MATLAB Function5 ==
  data: u1 input; u2 input; y output; Vpos_rail_dtg parameter
function y = and_cmos(u1, u2, Vpos_rail_dtg)

vth = Vpos_rail_dtg/2;

if (u1 > vth && u2 > vth)
    y = Vpos_rail_dtg;
else
    y = 0;
end

== matlab function dtmp_analysis/deadtime_generator_with_min_pulse_gen1/deadtime_minimum_pulse_rejction_generator_sm/minimum_pulse/MATLAB Function4 ==
  data: u1 input; u2 input; y output; Vpos_rail_dtg parameter
function y = and_cmos(u1, u2, Vpos_rail_dtg)

vth = Vpos_rail_dtg/2;

if (u1 > vth && u2 > vth)
    y = Vpos_rail_dtg;
else
    y = 0;
end

== matlab function dtmp_analysis/deadtime_generator_with_min_pulse_gen1/deadtime_minimum_pulse_rejction_generator_sm/minimum_pulse/MATLAB Function5 ==
  data: u1 input; u2 input; y output; Vpos_rail_dtg parameter
function y = and_cmos(u1, u2, Vpos_rail_dtg)

vth = Vpos_rail_dtg/2;

if (u1 > vth && u2 > vth)
    y = Vpos_rail_dtg;
else
    y = 0;
end

== matlab function dtmp_analysis/deadtime_generator_with_min_pulse_gen/deadtime_minimum_pulse_rejction_generator_sm1/minimum_pulse/MATLAB Function6 ==
  data: u input; y output; Vpos_rail_dtg parameter
function y = tschimitt_not_cmos(u, Vpos_rail_dtg)

persistent y_old

if isempty(y_old)
    y_old = 0;
end

vth1 = Vpos_rail_dtg*0.75;
vth2 = Vpos_rail_dtg*0.25;

if u > vth1
    y = 0;
    y_old = y;
elseif u < vth2
    y = Vpos_rail_dtg;
    y_old = y;
else
    y = y_old;
end

== matlab function dtmp_analysis/deadtime_generator_with_min_pulse_gen/deadtime_minimum_pulse_rejction_generator_sm1/minimum_pulse/MATLAB Function7 ==
  data: u input; y output; Vpos_rail_dtg parameter
function y = tschimitt_not_cmos(u, Vpos_rail_dtg)

persistent y_old

if isempty(y_old)
    y_old = 0;
end

vth1 = Vpos_rail_dtg*0.75;
vth2 = Vpos_rail_dtg*0.25;

if u > vth1
    y = 0;
    y_old = y;
elseif u < vth2
    y = Vpos_rail_dtg;
    y_old = y;
else
    y = y_old;
end

== matlab function dtmp_analysis/deadtime_generator_with_min_pulse_gen/deadtime_minimum_pulse_rejction_generator_sm1/minimum_pulse/MATLAB Function8 ==
  data: u input; y output; Vpos_rail_dtg parameter
function y = tschimitt_not_cmos(u, Vpos_rail_dtg)

persistent y_old

if isempty(y_old)
    y_old = 0;
end

vth1 = Vpos_rail_dtg*0.75;
vth2 = Vpos_rail_dtg*0.25;

if u > vth1
    y = 0;
    y_old = y;
elseif u < vth2
    y = Vpos_rail_dtg;
    y_old = y;
else
    y = y_old;
end

== matlab function dtmp_analysis/deadtime_generator_with_min_pulse_gen1/gate_cmds/MATLAB Function ==
  data: time input; y output; Ton_base parameter; dT_base parameter; vin_cmd parameter; N parameter
function y = fcn(time, Ton_base, dT_base, vin_cmd, N)
    y = 0;
    
    for n = 1:N
        if (time >= n*dT_base && time <= (n*dT_base + n*Ton_base))
            y = vin_cmd;
            break;
        end
    end
end

== matlab function dtmp_analysis/deadtime_generator_with_min_pulse_gen2/deadtime_minimum_pulse_rejction_generator_tchm/dead_time/MATLAB Function ==
  data: u input; y output; Vpos_rail_dtg parameter
function y = tschimitt_not_cmos(u, Vpos_rail_dtg)

persistent y_old

if isempty(y_old)
    y_old = 0;
end

vth1 = Vpos_rail_dtg*0.75;
vth2 = Vpos_rail_dtg*0.25;

if u > vth1
    y = 0;
    y_old = y;
elseif u < vth2
    y = Vpos_rail_dtg;
    y_old = y;
else
    y = y_old;
end

== matlab function dtmp_analysis/deadtime_generator_with_min_pulse_gen1/deadtime_minimum_pulse_rejction_generator_sm/dead_time/MATLAB Function7 ==
  data: u input; y output; Vpos_rail_dtg parameter
function y = tschimitt_not_cmos(u, Vpos_rail_dtg)

persistent y_old

if isempty(y_old)
    y_old = 0;
end

vth1 = Vpos_rail_dtg*0.75;
vth2 = Vpos_rail_dtg*0.25;

if u > vth1
    y = 0;
    y_old = y;
elseif u < vth2
    y = Vpos_rail_dtg;
    y_old = y;
else
    y = y_old;
end

== matlab function dtmp_analysis/deadtime_generator_with_min_pulse_gen2/deadtime_minimum_pulse_rejction_generator_tchm/dead_time/MATLAB Function1 ==
  data: u1 input; u2 input; y output; Vpos_rail_dtg parameter
function y = and_cmos(u1, u2, Vpos_rail_dtg)

vth = Vpos_rail_dtg/2;

if (u1 > vth && u2 > vth)
    y = Vpos_rail_dtg;
else
    y = 0;
end

== matlab function dtmp_analysis/deadtime_generator_with_min_pulse_gen2/deadtime_minimum_pulse_rejction_generator_tchm/dead_time/MATLAB Function2 ==
  data: u input; y output; Vpos_rail_dtg parameter
function y = tschimitt_not_cmos(u, Vpos_rail_dtg)

persistent y_old

if isempty(y_old)
    y_old = 0;
end

vth1 = Vpos_rail_dtg*0.75;
vth2 = Vpos_rail_dtg*0.25;

if u > vth1
    y = 0;
    y_old = y;
elseif u < vth2
    y = Vpos_rail_dtg;
    y_old = y;
else
    y = y_old;
end

== matlab function dtmp_analysis/deadtime_generator_with_min_pulse_gen2/deadtime_minimum_pulse_rejction_generator_tchm/dead_time/MATLAB Function3 ==
  data: u input; y output; Vpos_rail_dtg parameter
function y = tschimitt_not_cmos(u, Vpos_rail_dtg)

persistent y_old

if isempty(y_old)
    y_old = 0;
end

vth1 = Vpos_rail_dtg*0.75;
vth2 = Vpos_rail_dtg*0.25;

if u > vth1
    y = 0;
    y_old = y;
elseif u < vth2
    y = Vpos_rail_dtg;
    y_old = y;
else
    y = y_old;
end

== matlab function dtmp_analysis/deadtime_generator_with_min_pulse_gen2/deadtime_minimum_pulse_rejction_generator_tchm/dead_time/MATLAB Function4 ==
  data: u1 input; u2 input; y output; Vpos_rail_dtg parameter
function y = and_cmos(u1, u2, Vpos_rail_dtg)

vth = Vpos_rail_dtg/2;

if (u1 > vth && u2 > vth)
    y = Vpos_rail_dtg;
else
    y = 0;
end

== matlab function dtmp_analysis/deadtime_generator_with_min_pulse_gen2/deadtime_minimum_pulse_rejction_generator_tchm/dead_time/MATLAB Function5 ==
  data: u1 input; u2 input; y output; Vpos_rail_dtg parameter
function y = and_cmos(u1, u2, Vpos_rail_dtg)

vth = Vpos_rail_dtg/2;

if (u1 > vth && u2 > vth)
    y = Vpos_rail_dtg;
else
    y = 0;
end

== matlab function dtmp_analysis/deadtime_generator_with_min_pulse_gen2/deadtime_minimum_pulse_rejction_generator_tchm/dead_time/MATLAB Function6 ==
  data: u input; y output; Vpos_rail_dtg parameter
function y = tschimitt_not_cmos(u, Vpos_rail_dtg)

persistent y_old

if isempty(y_old)
    y_old = 0;
end

vth1 = Vpos_rail_dtg*0.75;
vth2 = Vpos_rail_dtg*0.25;

if u > vth1
    y = 0;
    y_old = y;
elseif u < vth2
    y = Vpos_rail_dtg;
    y_old = y;
else
    y = y_old;
end

== matlab function dtmp_analysis/deadtime_generator_with_min_pulse_gen2/deadtime_minimum_pulse_rejction_generator_tchm/dead_time/MATLAB Function7 ==
  data: u input; y output; Vpos_rail_dtg parameter
function y = tschimitt_not_cmos(u, Vpos_rail_dtg)

persistent y_old

if isempty(y_old)
    y_old = 0;
end

vth1 = Vpos_rail_dtg*0.75;
vth2 = Vpos_rail_dtg*0.25;

if u > vth1
    y = 0;
    y_old = y;
elseif u < vth2
    y = Vpos_rail_dtg;
    y_old = y;
else
    y = y_old;
end

== matlab function dtmp_analysis/deadtime_generator_with_min_pulse_gen2/deadtime_minimum_pulse_rejction_generator_tchm/dead_time/MATLAB Function8 ==
  data: u input; y output; Vpos_rail_dtg parameter
function y = tschimitt_not_cmos(u, Vpos_rail_dtg)

persistent y_old

if isempty(y_old)
    y_old = 0;
end

vth1 = Vpos_rail_dtg*0.75;
vth2 = Vpos_rail_dtg*0.25;

if u > vth1
    y = 0;
    y_old = y;
elseif u < vth2
    y = Vpos_rail_dtg;
    y_old = y;
else
    y = y_old;
end

== matlab function dtmp_analysis/deadtime_generator_with_min_pulse_gen2/deadtime_minimum_pulse_rejction_generator_tchm/dead_time/MATLAB Function9 ==
  data: u1 input; u2 input; y output; Vpos_rail_dtg parameter
function y = and_cmos(u1, u2, Vpos_rail_dtg)

vth = Vpos_rail_dtg/2;

if (u1 > vth && u2 > vth)
    y = Vpos_rail_dtg;
else
    y = 0;
end

== matlab function dtmp_analysis/deadtime_generator_with_min_pulse_gen2/deadtime_minimum_pulse_rejction_generator_tchm/minimum_pulse/MATLAB Function1 ==
  data: u1 input; u2 input; y output; Vpos_rail_dtg parameter
function y = and_cmos(u1, u2, Vpos_rail_dtg)

vth = Vpos_rail_dtg/2;

if (u1 > vth && u2 > vth)
    y = Vpos_rail_dtg;
else
    y = 0;
end

== matlab function dtmp_analysis/deadtime_generator_with_min_pulse_gen1/deadtime_minimum_pulse_rejction_generator_sm/dead_time/MATLAB Function3 ==
  data: u input; y output; Vpos_rail_dtg parameter
function y = tschimitt_not_cmos(u, Vpos_rail_dtg)

persistent y_old

if isempty(y_old)
    y_old = 0;
end

vth1 = Vpos_rail_dtg*0.75;
vth2 = Vpos_rail_dtg*0.25;

if u > vth1
    y = 0;
    y_old = y;
elseif u < vth2
    y = Vpos_rail_dtg;
    y_old = y;
else
    y = y_old;
end

== matlab function dtmp_analysis/deadtime_generator_with_min_pulse_gen2/deadtime_minimum_pulse_rejction_generator_tchm/minimum_pulse/MATLAB Function2 ==
  data: u input; y output; Vpos_rail_dtg parameter
function y = tschimitt_not_cmos(u, Vpos_rail_dtg)

persistent y_old

if isempty(y_old)
    y_old = 0;
end

vth1 = Vpos_rail_dtg*0.75;
vth2 = Vpos_rail_dtg*0.25;

if u > vth1
    y = 0;
    y_old = y;
elseif u < vth2
    y = Vpos_rail_dtg;
    y_old = y;
else
    y = y_old;
end

== matlab function dtmp_analysis/deadtime_generator_with_min_pulse_gen2/deadtime_minimum_pulse_rejction_generator_tchm/minimum_pulse/MATLAB Function3 ==
  data: u input; y output; Vpos_rail_dtg parameter
function y = tschimitt_not_cmos(u, Vpos_rail_dtg)

persistent y_old

if isempty(y_old)
    y_old = 0;
end

vth1 = Vpos_rail_dtg*0.75;
vth2 = Vpos_rail_dtg*0.25;

if u > vth1
    y = 0;
    y_old = y;
elseif u < vth2
    y = Vpos_rail_dtg;
    y_old = y;
else
    y = y_old;
end

== matlab function dtmp_analysis/deadtime_generator_with_min_pulse_gen2/deadtime_minimum_pulse_rejction_generator_tchm/minimum_pulse/MATLAB Function4 ==
  data: u1 input; u2 input; y output; Vpos_rail_dtg parameter
function y = and_cmos(u1, u2, Vpos_rail_dtg)

vth = Vpos_rail_dtg/2;

if (u1 > vth && u2 > vth)
    y = Vpos_rail_dtg;
else
    y = 0;
end

== matlab function dtmp_analysis/deadtime_generator_with_min_pulse_gen2/deadtime_minimum_pulse_rejction_generator_tchm/minimum_pulse/MATLAB Function5 ==
  data: u1 input; u2 input; y output; Vpos_rail_dtg parameter
function y = and_cmos(u1, u2, Vpos_rail_dtg)

vth = Vpos_rail_dtg/2;

if (u1 > vth && u2 > vth)
    y = Vpos_rail_dtg;
else
    y = 0;
end

== matlab function dtmp_analysis/deadtime_generator_with_min_pulse_gen2/deadtime_minimum_pulse_rejction_generator_tchm/minimum_pulse/MATLAB Function6 ==
  data: u input; y output; Vpos_rail_dtg parameter
function y = tschimitt_not_cmos(u, Vpos_rail_dtg)

persistent y_old

if isempty(y_old)
    y_old = 0;
end

vth1 = Vpos_rail_dtg*0.75;
vth2 = Vpos_rail_dtg*0.25;

if u > vth1
    y = 0;
    y_old = y;
elseif u < vth2
    y = Vpos_rail_dtg;
    y_old = y;
else
    y = y_old;
end

== matlab function dtmp_analysis/deadtime_generator_with_min_pulse_gen2/deadtime_minimum_pulse_rejction_generator_tchm/minimum_pulse/MATLAB Function7 ==
  data: u input; y output; Vpos_rail_dtg parameter
function y = tschimitt_not_cmos(u, Vpos_rail_dtg)

persistent y_old

if isempty(y_old)
    y_old = 0;
end

vth1 = Vpos_rail_dtg*0.75;
vth2 = Vpos_rail_dtg*0.25;

if u > vth1
    y = 0;
    y_old = y;
elseif u < vth2
    y = Vpos_rail_dtg;
    y_old = y;
else
    y = y_old;
end

== matlab function dtmp_analysis/deadtime_generator_with_min_pulse_gen2/deadtime_minimum_pulse_rejction_generator_tchm/minimum_pulse/MATLAB Function8 ==
  data: u input; y output; Vpos_rail_dtg parameter
function y = tschimitt_not_cmos(u, Vpos_rail_dtg)

persistent y_old

if isempty(y_old)
    y_old = 0;
end

vth1 = Vpos_rail_dtg*0.75;
vth2 = Vpos_rail_dtg*0.25;

if u > vth1
    y = 0;
    y_old = y;
elseif u < vth2
    y = Vpos_rail_dtg;
    y_old = y;
else
    y = y_old;
end

== matlab function dtmp_analysis/deadtime_generator_with_min_pulse_gen2/gate_cmds/MATLAB Function ==
  data: time input; y output; Ton_base parameter; dT_base parameter; vin_cmd parameter; N parameter
function y = fcn(time, Ton_base, dT_base, vin_cmd, N)
    y = 0;
    
    for n = 1:N
        if (time >= n*dT_base && time <= (n*dT_base + n*Ton_base))
            y = vin_cmd;
            break;
        end
    end
end

== matlab function dtmp_analysis/deadtime_generator_with_min_pulse_gen1/deadtime_minimum_pulse_rejction_generator_sm/dead_time/MATLAB Function8 ==
  data: u input; y output; Vpos_rail_dtg parameter
function y = tschimitt_not_cmos(u, Vpos_rail_dtg)

persistent y_old

if isempty(y_old)
    y_old = 0;
end

vth1 = Vpos_rail_dtg*0.75;
vth2 = Vpos_rail_dtg*0.25;

if u > vth1
    y = 0;
    y_old = y;
elseif u < vth2
    y = Vpos_rail_dtg;
    y_old = y;
else
    y = y_old;
end

== matlab function dtmp_analysis/deadtime_generator_with_min_pulse_gen1/deadtime_minimum_pulse_rejction_generator_sm/minimum_pulse/MATLAB Function3 ==
  data: u input; y output; Vpos_rail_dtg parameter
function y = tschimitt_not_cmos(u, Vpos_rail_dtg)

persistent y_old

if isempty(y_old)
    y_old = 0;
end

vth1 = Vpos_rail_dtg*0.75;
vth2 = Vpos_rail_dtg*0.25;

if u > vth1
    y = 0;
    y_old = y;
elseif u < vth2
    y = Vpos_rail_dtg;
    y_old = y;
else
    y = y_old;
end

== matlab function dtmp_analysis/deadtime_generator_with_min_pulse_gen1/deadtime_minimum_pulse_rejction_generator_sm/minimum_pulse/MATLAB Function2 ==
  data: u input; y output; Vpos_rail_dtg parameter
function y = tschimitt_not_cmos(u, Vpos_rail_dtg)

persistent y_old

if isempty(y_old)
    y_old = 0;
end

vth1 = Vpos_rail_dtg*0.75;
vth2 = Vpos_rail_dtg*0.25;

if u > vth1
    y = 0;
    y_old = y;
elseif u < vth2
    y = Vpos_rail_dtg;
    y_old = y;
else
    y = y_old;
end

== matlab function dtmp_analysis/deadtime_generator_with_min_pulse_gen1/deadtime_minimum_pulse_rejction_generator_sm/minimum_pulse/MATLAB Function6 ==
  data: u input; y output; Vpos_rail_dtg parameter
function y = tschimitt_not_cmos(u, Vpos_rail_dtg)

persistent y_old

if isempty(y_old)
    y_old = 0;
end

vth1 = Vpos_rail_dtg*0.75;
vth2 = Vpos_rail_dtg*0.25;

if u > vth1
    y = 0;
    y_old = y;
elseif u < vth2
    y = Vpos_rail_dtg;
    y_old = y;
else
    y = y_old;
end

== matlab function dtmp_analysis/deadtime_generator_with_min_pulse_gen1/deadtime_minimum_pulse_rejction_generator_sm/minimum_pulse/MATLAB Function8 ==
  data: u input; y output; Vpos_rail_dtg parameter
function y = tschimitt_not_cmos(u, Vpos_rail_dtg)

persistent y_old

if isempty(y_old)
    y_old = 0;
end

vth1 = Vpos_rail_dtg*0.75;
vth2 = Vpos_rail_dtg*0.25;

if u > vth1
    y = 0;
    y_old = y;
elseif u < vth2
    y = Vpos_rail_dtg;
    y_old = y;
else
    y = y_old;
end

== matlab function dtmp_analysis/deadtime_generator_with_min_pulse_gen1/deadtime_minimum_pulse_rejction_generator_sm/minimum_pulse/MATLAB Function7 ==
  data: u input; y output; Vpos_rail_dtg parameter
function y = tschimitt_not_cmos(u, Vpos_rail_dtg)

persistent y_old

if isempty(y_old)
    y_old = 0;
end

vth1 = Vpos_rail_dtg*0.75;
vth2 = Vpos_rail_dtg*0.25;

if u > vth1
    y = 0;
    y_old = y;
elseif u < vth2
    y = Vpos_rail_dtg;
    y_old = y;
else
    y = y_old;
end

== matlab function dtmp_analysis/deadtime_generator_with_min_pulse_gen/gate_cmds/MATLAB Function ==
  data: time input; y output; Ton_base parameter; dT_base parameter; vin_cmd parameter; N parameter
function y = fcn(time, Ton_base, dT_base, vin_cmd, N)
    y = 0;
    
    for n = 1:N
        if (time >= n*dT_base && time <= (n*dT_base + n*Ton_base))
            y = vin_cmd;
            break;
        end
    end
end
